simulink model "Bsw_DCAC"  (R2023b)
settings: Solver=ode3  StartTime=0.0  StopTime=inf  RelTol=1e-3
settings Model: Creator=VanillaC  LastModifiedBy=VanillaC
settings OptimizationCC: DefaultParameterBehavior=Inlined  EnhancedBackFolding=on  PassReuseOutputArgsAs=Individual arguments  ZeroExternalMemoryAtStartup=off  ZeroInternalMemoryAtStartup=off  OptimizeBlockOrder=speed  DifferentSizesBufferReuse=on  OptimizationCustomize=off  EfficientTunableParamExpr=on
settings DebuggingCC: ParameterTunabilityLossMsg=error
settings SFSimCC: MATLABDynamicMemAlloc=off
settings RTWCC: Description=Embedded Coder  SystemTargetFile=ert.tlc  TemplateMakefile=ert_default_tmf
settings CodeAppCC: ForceParamTrailComments=on  IgnoreCustomStorageClasses=off  OperatorAnnotations=on  SimulinkDataObjDesc=on  SFDataObjDesc=on  InsertBlockDesc=on
settings ERTTargetCC: TargetLangStandard=C99 (ISO)  GenerateSampleERTMain=on  InlinedParameterPlacement=NonHierarchical  ERTCustomFileTemplate=example_file_process.tlc

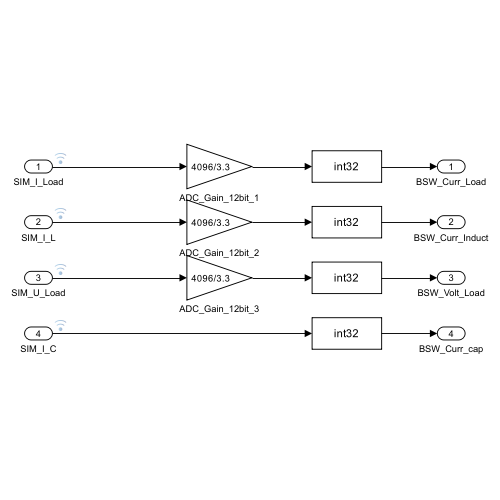
[thumbnail: Simulink's stored preview of the top-level diagram]
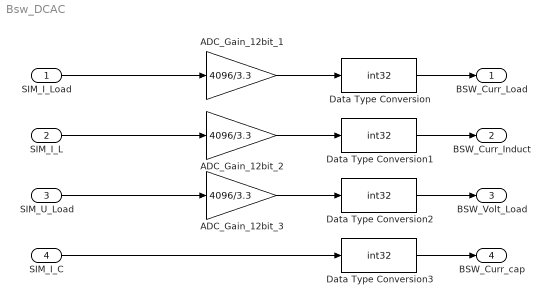
== system Bsw_DCAC ==
  SIM_I_Load : Inport  OutDataTypeStr=single
  SIM_I_L : Inport  Port=2  OutDataTypeStr=single
  SIM_U_Load : Inport  Port=3  OutDataTypeStr=single
  SIM_I_C : Inport  Port=4  OutDataTypeStr=single
  ADC_Gain_12bit_1 : Gain  Gain=4096/3.3
  ADC_Gain_12bit_2 : Gain  Gain=4096/3.3
  ADC_Gain_12bit_3 : Gain  Gain=4096/3.3
  Data Type Conversion{,1..3} (4 alike) : DataTypeConversion  OutDataTypeStr=int32  SaturateOnIntegerOverflow=off  RndMeth=Floor
  BSW_Curr_Load : Outport
  BSW_Curr_Induct : Outport  Port=2
  BSW_Volt_Load : Outport  Port=3
  BSW_Curr_cap : Outport  Port=4
  wires:
  SIM_I_C/1 -> Data Type Conversion3/1
  Data Type Conversion/1 -> BSW_Curr_Load/1
  ADC_Gain_12bit_1/1 -> Data Type Conversion/1
  SIM_I_Load/1 -> ADC_Gain_12bit_1/1
  Data Type Conversion1/1 -> BSW_Curr_Induct/1
  ADC_Gain_12bit_2/1 -> Data Type Conversion1/1
  SIM_I_L/1 -> ADC_Gain_12bit_2/1
  ADC_Gain_12bit_3/1 -> Data Type Conversion2/1
  SIM_U_Load/1 -> ADC_Gain_12bit_3/1
  Data Type Conversion2/1 -> BSW_Volt_Load/1
  Data Type Conversion3/1 -> BSW_Curr_cap/1
